simulink model "TopModel"  (R2019b)
settings: Solver=VariableStepAuto  StartTime=0.0  StopTime=10.0  RelTol=1e-3  EnableMultiTasking=on
settings Model: Creator=The MathWorks, Inc.  LastModifiedBy=clement.hamel
settings DataIOCC: LimitDataPoints=on  ReturnWorkspaceOutputs=off
settings OptimizationCC: LifeSpan=inf
settings DebuggingCC: AllowSymbolicDim=off  SFUnexpectedBacktrackingDiag=warning  SFNoUnconditionalDefaultTransitionDiag=warning  SFExecutionAtInitializationDiag=none  ArithmeticOperatorsInVariantConditions=warning
settings ModelReferenceCC: PropagateSignalLabelsOutOfModel=off
settings SFSimCC: SimUseLocalCustomCode=off  CustomCodeUndefinedFunction=UseInterfaceOnly
settings RTWCC: RTWUseLocalCustomCode=off
settings CodeAppCC: StateflowObjectComments=on
settings GRTTargetCC: TargetLangStandard=C89/C90 (ANSI)
settings ConfigComp: CovMetricSettings=dw  CovHtmlReporting=on  CovSaveCumulativeToWorkspaceVar=on  CovSaveSingleToWorkspaceVar=on  CovExternalEMLEnable=off

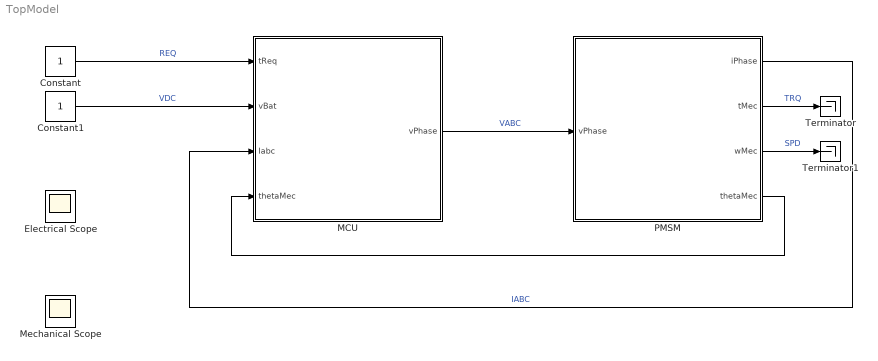
== system TopModel ==
  Constant : Constant
  Constant1 : Constant
  Electrical Scope : Scope
      settings: Floating=on
  MCU : Subsystem
  Mechanical Scope : Scope
      settings: Floating=on
  PMSM : Subsystem
  Terminator : Terminator
  Terminator1 : Terminator
  wires:
  Constant1/1 -> MCU/2(vBat)  "VDC"
  PMSM/4(thetaMec) -> MCU/4(thetaMec)
  MCU/1(vPhase) -> PMSM/1(vPhase)  "VABC"
  PMSM/1(iPhase) -> MCU/3(Iabc)  "IABC"
  Constant/1 -> MCU/1(tReq)  "REQ"
  PMSM/2(tMec) -> Terminator/1  "TRQ"
  PMSM/3(wMec) -> Terminator1/1  "SPD"

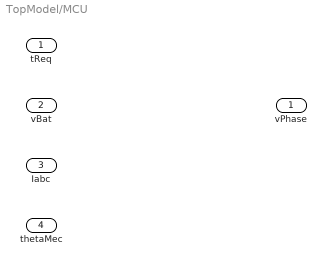
== system TopModel/MCU ==
  tReq : Inport
  vBat : Inport  Port=2
  Iabc : Inport  Port=3
  thetaMec : Inport  Port=4
  vPhase : Outport

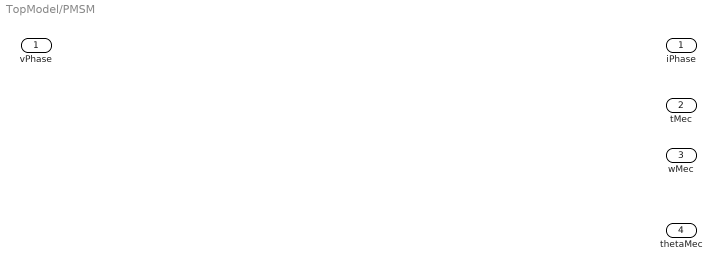
== system TopModel/PMSM ==
  vPhase : Inport
  iPhase : Outport
  tMec : Outport  Port=2
  wMec : Outport  Port=3
  thetaMec : Outport  Port=4
